simulink model "blackbanana_kinlam_ver2"  (R2022b)
settings: Solver=VariableStepAuto  StartTime=0.0  StopTime=20  RelTol=1e-3
model workspace: external: MAT-File params.mat (data not in the file)
undefined symbols (not defined in the file): lambda_allocated_memory, lambda_parallel_instances
libraries: VACLib x2
settings Model: Creator=KarlO  LastModifiedBy=KarlO

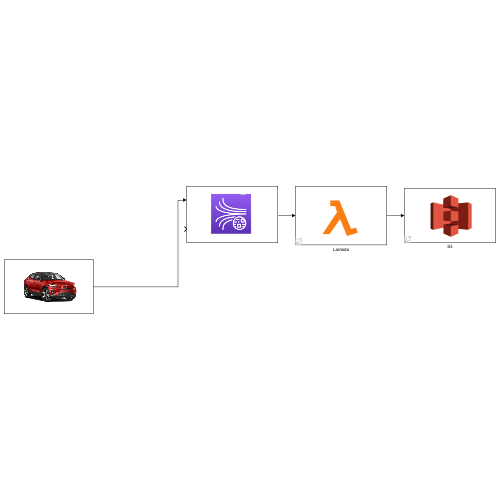
[thumbnail: Simulink's stored preview of the top-level diagram]
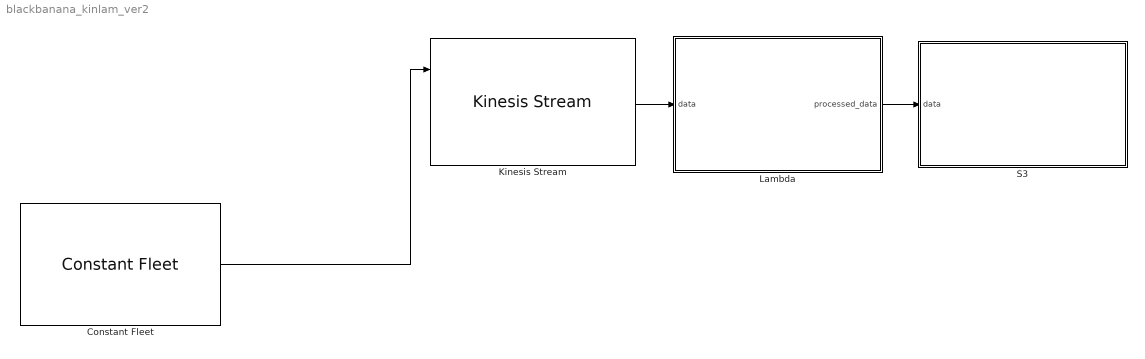
== system blackbanana_kinlam_ver2 ==
  Constant Fleet : VACLib/Vehicle Components/Constant Fleet  SystemSampleTime=-1  VariantActivationTime=update diagram  Latency=0  AutoFrameSizeCalculation=off
      settings: SourceProductName=Volvo Architechture Components
  Kinesis Stream : VACLib/AWS Components/Kinesis Stream  SystemSampleTime=-1  VariantActivationTime=update diagram  Latency=0  AutoFrameSizeCalculation=off
      settings: SourceProductName=Volvo Architechture Components
  Lambda : Subsystem  AncestorBlock=VACLib/AWS Components/Lambda
      settings: LibrarySourceBlock=VACLib/AWS Components/Lambda
      mask Display: image('C:\Users\KarlO\architectural-tradeoff-analysis\DCA-simulator\Volvo Architecture\VAC library\Images\VAC\aws-lambda-1.svg',[60,20,80,80]); % Use "Edit Image" on toolstrip to change.
  S3 : Subsystem  AncestorBlock=VACLib/AWS Components/S3
      settings: LibrarySourceBlock=VACLib/AWS Components/S3
      mask Display: image('C:\Users\KarlO\architectural-tradeoff-analysis\DCA-simulator\Volvo Architecture\VAC library\Images\VAC\Amazon-S3-Logo.svg',[55,10,100,100]); % Use "Edit Image" on toolstrip to change.
  wires:
  Kinesis Stream/1 -> Lambda/1(data)
  Lambda/1(processed_data) -> S3/1(data)
  Constant Fleet/1 -> Kinesis Stream/1

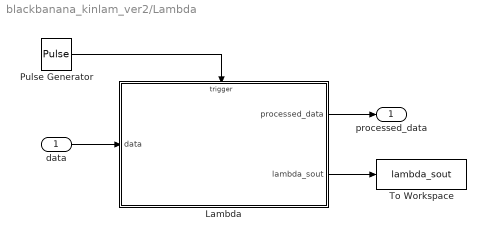
== system blackbanana_kinlam_ver2/Lambda ==
  data : Inport
  Lambda : MATLAB Function  TreatAsAtomicUnit=on
  Pulse Generator : DiscretePulseGenerator  PulseType=Time based  Period=1/log10(lambda_allocated_memory)  PulseWidth=5
  To Workspace : ToWorkspace  VariableName=lambda_sout  SaveFormat=Timeseries  SampleTime=-1
  processed_data : Outport
  wires:
  Lambda/1(processed_data) -> processed_data/1
  Lambda/2(lambda_sout) -> To Workspace/1
  data/1 -> Lambda/1(data)
  Pulse Generator/1 -> Lambda/Trigger

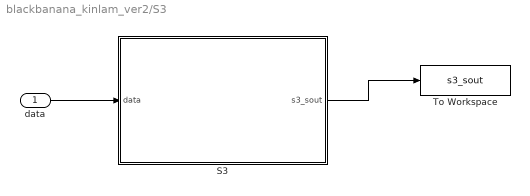
== system blackbanana_kinlam_ver2/S3 ==
  data : Inport
  S3 : MATLAB Function  TreatAsAtomicUnit=on
  To Workspace : ToWorkspace  VariableName=s3_sout  SaveFormat=Timeseries  SampleTime=-1
  wires:
  data/1 -> S3/1(data)
  S3/1(s3_sout) -> To Workspace/1

== matlab function blackbanana_kinlam_ver2/Lambda/Lambda ==
  data: processed_data output; data input; lambda_sout output; lambda_parallel_instances parameter; lambda_allocated_memory parameter
  events: clock input RISING_EDGE_EVENT
function [processed_data,lambda_sout]= lambda(data, lambda_parallel_instances, lambda_allocated_memory)
%Price of lambda instance depends on memory allocated to it
%An increase in memory size triggers an equivalent increase in CPU available to your function.

% Data left in lambda queue to process
persistent remaining_data;
% Chunk size on incoming data
persistent chunk_size;
% Previously received to detect change in incoming data
persistent prev_received;

% Output variables
persistent lambda_cost;
persistent lambda_latency;

%Limited for 1 to be divisible by computation time 1/x = even
computation_time = 1/log10(lambda_allocated_memory);

if isempty(remaining_data)
    remaining_data = 0;
    prev_received = 0;
    lambda_latency = 0;
    lambda_cost = 0;
end

% Get new data - 0 if no change
new_data = max(0,data(1) - prev_received);
prev_received = prev_received + new_data;
remaining_data = remaining_data + new_data;
chunk_size = data(2);

chunks_to_process = floor(lambda_allocated_memory / chunk_size);
effective_size_processed = (chunks_to_process*chunk_size);

% How many lambda computations is left on currently remaining data
computations_left = remaining_data / effective_size_processed;

if remaining_data > 0
    % Get max number of possible computations if computations left is
    % higher than what can be done in one go 
    computations = min(lambda_parallel_instances,computations_left);

    % Subtract data to be processed
    remaining_data = remaining_data - (computations * effective_size_processed);

    % Calculate memory size needed for lambda
    allocated_memory = lambda_allocated_memory;

    % Calculate lambda pricing

    % GB capacity in parallel
    configured_concurr = lambda_parallel_instances*(allocated_memory/1000);
    % GB seconds used
    provisioned_concurr = configured_concurr * 0.2;
    % $0.0000041667 per GBs
    concurr_cost = provisioned_concurr * 0.0000041667;
    % $0.2 per 1M requests
    request_cost = (computations/1000000) * 0.2;

    % Record cost
    lambda_cost = lambda_cost + concurr_cost + request_cost;

    if remaining_data > 0 
        lambda_latency = max(lambda_latency, (remaining_data/(effective_size_processed*computations))*computation_time);
    end
end

processed_data = [prev_received-remaining_data, data(2), data(3), data(4)];
lambda_sout = [lambda_latency, lambda_cost, 0,0];

== matlab function blackbanana_kinlam_ver2/S3/S3 ==
  data: data input; s3_sout output
function s3_sout = S3(data)

% Keeps count of amount of data buckets (MB)
persistent in_storage;
% Overall cost for usage
persistent s3_cost;

if isempty(in_storage)
    in_storage = 0;
    s3_cost = 0;
end

% Received data (Might be zero if read in between pulses)
% data_packets = (size_sent_in_total, size_of_each_file)
new_data = max(0,data(1) - in_storage);
in_storage = in_storage + new_data;
chunk_size = data(2);

if (new_data > 0)
    % Count packets
    no_of_packets = chunk_size/new_data;
    % Upfront cost ($0.005 per 1000 PUT)
    s3_cost = s3_cost + no_of_packets*0.000005;
end

% [latency, cost, reliability, scalability]
s3_sout = [0, s3_cost,0,0];
